simulink model "testAlphaFloor"  (R2013b)
settings: Solver=VariableStepDiscrete  StartTime=0.0  StopTime=10  RelTol=1e-3
libraries: carnot x3, simulink x1
settings Model: Creator=drhf  LastModifiedBy=drhf
settings DataIOCC: ReturnWorkspaceOutputs=on
settings OptimizationCC: InlineParams=on
settings DebuggingCC: ReadBeforeWriteMsg=DisableAll  WriteAfterWriteMsg=DisableAll  WriteAfterReadMsg=DisableAll  MultiTaskDSMMsg=none
settings ModelReferenceCC: UpdateModelReferenceTargets=IfOutOfDate
settings SFSimCC: SFSimEcho=off

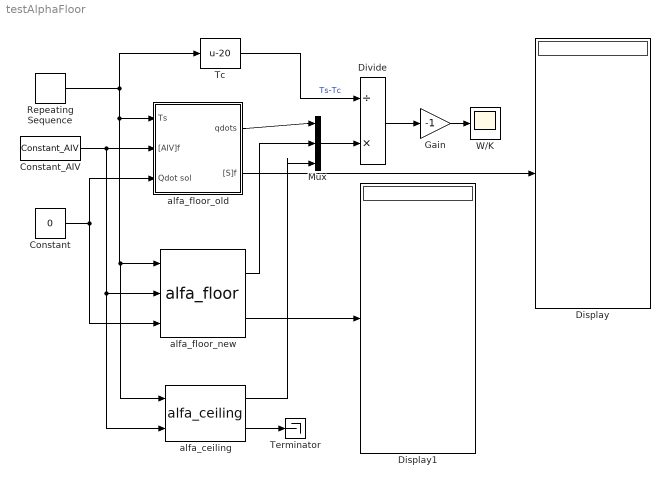
== system testAlphaFloor ==
  Constant : Constant  Value=0
  Constant_AIV : carnot/Source/Ventilation/Constant_AIV  Tsens=20  Tcon=20  Trad=20  mw=0.012  mco=0.01  rhoair=1.2  cpair=1004  pair=100000  nair=0.5
  Display : Display
  Display1 : Display
  Divide : Product  Inputs=/*
  Gain : Gain  Gain=-1
  Mux : Mux  Inputs=3
  Repeating Sequence : simulink/Sources/Repeating Sequence  rep_seq_t=[0 10]  rep_seq_y=[10 30]
  Tc : Bias  Bias=-20
  Terminator : Terminator
  W/K : Scope
  alfa_ceiling : carnot/Load/Houses/heat_transfer/alfa_ceiling  active=0  emission_c=0.65  wallsurface=1
  alfa_floor_new : carnot/Load/Houses/heat_transfer/alfa_floor  active=0  emission_f=0.65  wallsurface=1
  alfa_floor_old : Subsystem  AncestorBlock=carnot/Load/Houses/heat_transfer/alfa_floor  mask(ALFA){active=0, emission_f=0.65, wallsurface=1}
      mask prompts: active "active layer (0 / 1)"; emission_f "Longwave emissivity of surface (0..1)"; wallsurface "Floor surface in m²"
      mask help:
      | Convective and radiative heat transfer at the SURFACE OF A HORIZONTAL FLOOR.
      |
      | [AIV] : conditions of zone node,
      | Ts : temperature of wall surface, °C,
      | qdots : specific heat flow into wall construction, W/m^2,
      | [S] : heat and air flow to zone node.
  wires:
  Constant_AIV/1 -> alfa_ceiling/2, alfa_floor_new/2, alfa_floor_old/2("[AIV]f")
  Repeating Sequence/1 -> Tc/1, alfa_ceiling/1, alfa_floor_new/1, alfa_floor_old/1(Ts)
  alfa_floor_old/2("[S]f") -> Display/1
  alfa_floor_new/2 -> Display1/1
  Constant/1 -> alfa_floor_new/3, alfa_floor_old/3(Qdot sol)
  alfa_floor_old/1(qdots) -> Mux/1
  alfa_floor_new/1 -> Mux/2
  Mux/1 -> Divide/2
  Divide/1 -> Gain/1
  Tc/1 -> Divide/1  "Ts-Tc"
  alfa_ceiling/2 -> Terminator/1
  Gain/1 -> W/K/1
  alfa_ceiling/1 -> Mux/3

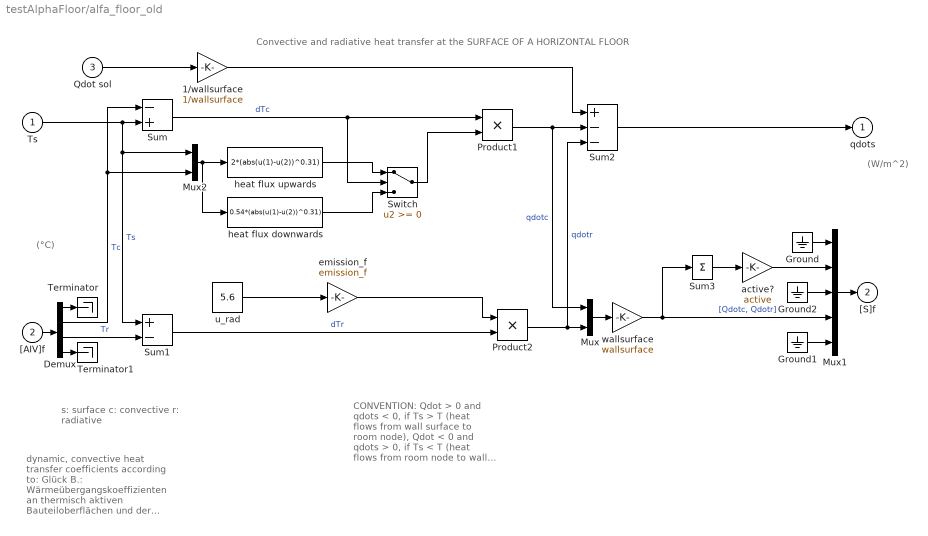
== system testAlphaFloor/alfa_floor_old ==
  note: dynamic, convective heat transfer coefficients according to: Glück B.: Wärmeübergangskoeffizienten an thermisch aktiven Bauteiloberflächen
      | und der Übergang zu Basiskennlinien für die Wärmestromdichte; gi Gesundheits-Ingenieur; 128. Jahrgang 2007, Heft 1, Seiten 1-10
  note: (°C)
  note: (W/m^2)
  note: Convective and radiative heat transfer at the SURFACE OF A HORIZONTAL FLOOR
  note: s: surface
      | c: convective
      | r: radiative
  note: CONVENTION:
      | Qdot > 0 and qdots < 0, if Ts > T (heat flows from wall surface to room node),
      | Qdot < 0 and qdots > 0, if Ts < T (heat flows from room node to wall surface).
  Ts : Inport
  "[AIV]f" : Inport  Port=2
  Qdot sol : Inport  Port=3
  1/wallsurface : Gain  Gain=1/wallsurface  SaturateOnIntegerOverflow=on  OutDataTypeStr=Inherit: Same as input  ParamDataTypeStr=Inherit: Same as input
  Demux : Demux  Outputs=[1 1 1 6]
  Ground : Ground
  Ground1 : Ground
  Ground2 : Ground
  Mux : Mux  Inputs=[1 1]
  Mux1 : Mux  Inputs=[4 1 1 2 5]
  Mux2 : Mux  Inputs=2
  Product1 : Product  SaturateOnIntegerOverflow=on  RndMeth=Zero  InputSameDT=on  OutDataTypeStr=Inherit: Same as first input
  Product2 : Product  SaturateOnIntegerOverflow=on  RndMeth=Zero  InputSameDT=on  OutDataTypeStr=Inherit: Same as first input
  Sum : Sum  Inputs=-+  SaturateOnIntegerOverflow=on  InputSameDT=on  OutDataTypeStr=Inherit: Same as first input
  Sum1 : Sum  Inputs=+-  SaturateOnIntegerOverflow=on  InputSameDT=on  OutDataTypeStr=Inherit: Same as first input
  Sum2 : Sum  Inputs=+--  SaturateOnIntegerOverflow=on  InputSameDT=on  OutDataTypeStr=Inherit: Same as first input
  Sum3 : Sum  Inputs=1  SaturateOnIntegerOverflow=on  InputSameDT=on  OutDataTypeStr=Inherit: Same as first input
  Switch : Switch
  Terminator : Terminator
  Terminator1 : Terminator
  active? : Gain  Gain=active  SaturateOnIntegerOverflow=on  OutDataTypeStr=Inherit: Same as input  ParamDataTypeStr=Inherit: Same as input
  emission_f : Gain  Gain=emission_f  SaturateOnIntegerOverflow=on  OutDataTypeStr=Inherit: Same as input  ParamDataTypeStr=Inherit: Same as input
  heat flux downwards : Fcn  Expr=0.54*(abs(u(1)-u(2))^0.31)
  heat flux upwards : Fcn  Expr=2*(abs(u(1)-u(2))^0.31)
  u_rad : Constant  Value=5.6
  wallsurface : Gain  Gain=wallsurface  SaturateOnIntegerOverflow=on  OutDataTypeStr=Inherit: Same as input  ParamDataTypeStr=Inherit: Same as input
  qdots : Outport
  "[S]f" : Outport  Port=2
  wires:
  heat flux downwards/1 -> Switch/3
  heat flux upwards/1 -> Switch/1
  Switch/1 -> Product1/2
  Mux2/1 -> heat flux downwards/1, heat flux upwards/1
  Demux/3 -> Sum1/2  "Tr"
  Product1/1 -> Sum2/2, Mux/1  "qdotc"
  Sum/1 -> Switch/2, Product1/1  "dTc"
  Mux/1 -> wallsurface/1
  Product2/1 -> Sum2/3, Mux/2  "qdotr"
  u_rad/1 -> emission_f/1
  emission_f/1 -> Product2/1
  Sum1/1 -> Product2/2  "dTr"
  Demux/1 -> Terminator/1
  "[AIV]f"/1 -> Demux/1
  Demux/4 -> Terminator1/1
  1/wallsurface/1 -> Sum2/1
  Ts/1 -> Mux2/1, Sum1/1, Sum/2  "Ts"
  Sum2/1 -> qdots/1
  Demux/2 -> Mux2/2, Sum/1  "Tc"
  wallsurface/1 -> Mux1/4, Sum3/1  "[Qdotc, Qdotr]"
  Qdot sol/1 -> 1/wallsurface/1
  Sum3/1 -> active?/1
  Ground/1 -> Mux1/1
  Ground1/1 -> Mux1/5
  Mux1/1 -> "[S]f"/1
  Ground2/1 -> Mux1/3
  active?/1 -> Mux1/2
